simulink model "radar_lidar_road_double"  (R2021b)
settings: Solver=FixedStepDiscrete  StartTime=0.0  StopTime=10.0  RelTol=1e-3
model workspace (MAT data in the model file):
  firstWarning = 1
  originalScenarioChecksum = '4A544F35B5F16CEB30B2C31E0C92B54A'
libraries: drivingscenarioandsensors x4
(part 2 of 34)

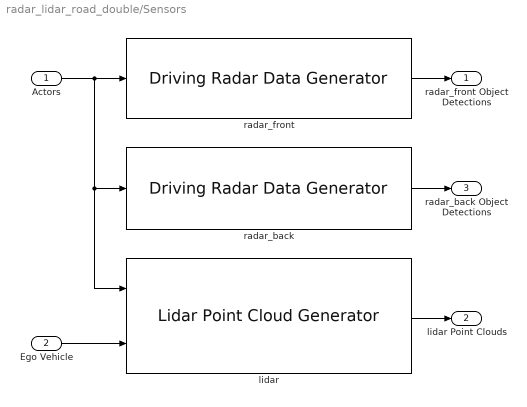
== system radar_lidar_road_double/Sensors ==
  Actors : Inport
  Ego Vehicle : Inport  Port=2
  lidar : drivingscenarioandsensors/Lidar Point Cloud Generator  SensorIndex=2  UpdateInterval=0.1  SensorLocation=[0.05 0]  Height=1.6  Yaw=0  Pitch=0  Roll=30  DetectionCoordinates=Ego Cartesian  HasEgoVehicle=on  EgoVehicleActorID=2  HasRoadsInputPort=on  ActorProfilesSource=From Scenario Reader block  ActorProfilesVariableName=actor_profiles  MaxRange=120  RangeAccuracy=0.002  AzimuthResolution=0.16  ElevationResolution=1.25  AzimuthLimits=[-180 180]  ElevationLimits=[-20 20]  HasNoise=on
      settings: SourceProductBaseCode=DR
